simulink model "NewtonRaphson"  (R2018b)
settings: Solver=FixedStepAuto  StartTime=0.0  StopTime=10.0  FixedStep=1  RelTol=1e-3
undefined symbols (not defined in the file or in its folder): a, b, c
libraries: simulink x8, hdlsllib x3
settings Model: Creator=meyer  LastModifiedBy=meyer

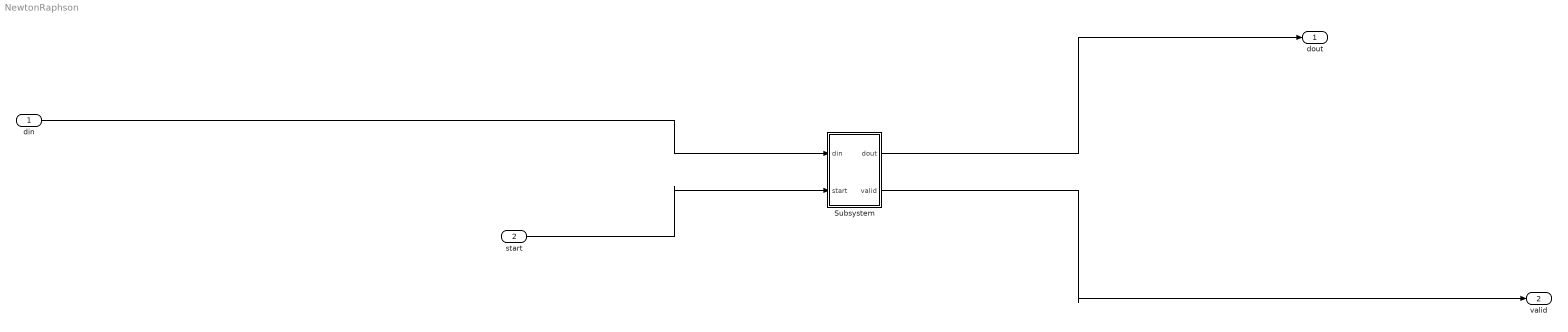
== system NewtonRaphson ==
  din : Inport  OutDataTypeStr=fixdt(1,32,16)
  start : Inport  Port=2  OutDataTypeStr=boolean
  Subsystem : Subsystem
  dout : Outport
  valid : Outport  Port=2
  wires:
  din/1 -> Subsystem/1(din)
  start/1 -> Subsystem/2(start)
  Subsystem/1(dout) -> dout/1
  Subsystem/2(valid) -> valid/1

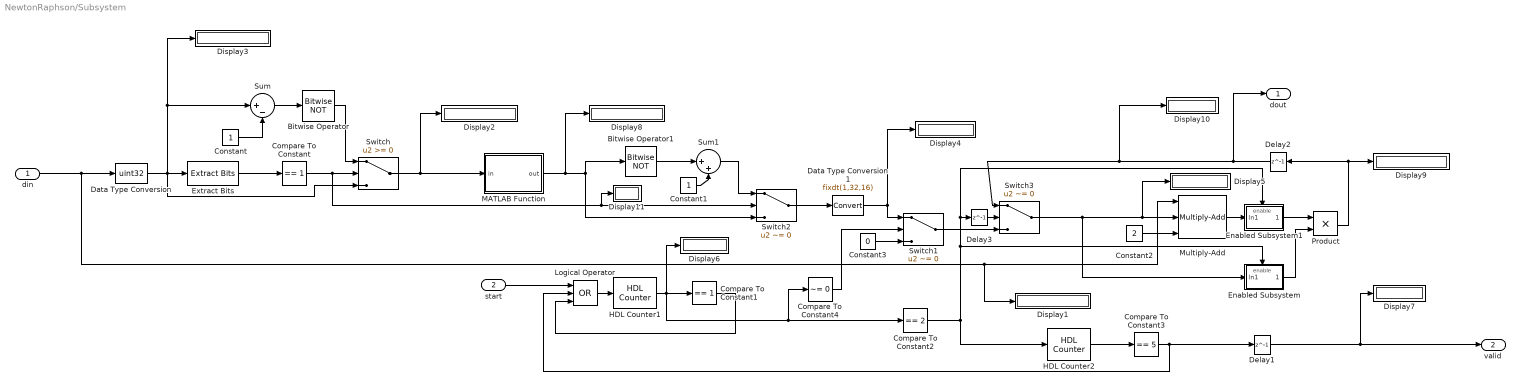
== system NewtonRaphson/Subsystem ==
  din : Inport  OutDataTypeStr=fixdt(1,32,16)
  start : Inport  Port=2  OutDataTypeStr=boolean
  Bitwise Operator : simulink/Logic and Bit Operations/Bitwise Operator  logicop=NOT  UseBitMask=off  BitMask=bin2dec('11011001')  BitMaskRealWorld=Stored Integer
  Bitwise Operator1 : simulink/Logic and Bit Operations/Bitwise Operator  logicop=NOT  UseBitMask=off  BitMask=bin2dec('11011001')  BitMaskRealWorld=Stored Integer
  Compare To Constant : simulink/Logic and Bit Operations/Compare To Constant  relop===  const=1  OutDataTypeStr=boolean
  Compare To Constant1 : simulink/Logic and Bit Operations/Compare To Constant  relop===  const=1  OutDataTypeStr=boolean
  Compare To Constant2 : simulink/Logic and Bit Operations/Compare To Constant  relop===  const=2  OutDataTypeStr=boolean
  Compare To Constant3 : simulink/Logic and Bit Operations/Compare To Constant  relop===  const=5  OutDataTypeStr=boolean
  Compare To Constant4 : simulink/Logic and Bit Operations/Compare To Constant  relop=~=  const=0  OutDataTypeStr=boolean
  Constant : Constant  OutDataTypeStr=uint32  SampleTime=-1
  Constant1 : Constant  OutDataTypeStr=uint32  SampleTime=-1
  Constant2 : Constant  Value=2  OutDataTypeStr=fixdt(1,32,16)  SampleTime=-1
  Constant3 : Constant  Value=0  OutDataTypeStr=fixdt(1,32,16)  SampleTime=-1
  Data Type Conversion : DataTypeConversion  OutDataTypeStr=uint32  ConvertRealWorld=Stored Integer (SI)
  Data Type Conversion1 : DataTypeConversion  OutDataTypeStr=fixdt(1,32,16)  ConvertRealWorld=Stored Integer (SI)
  Delay1 : Delay  DelayLength=1
  Delay2 : Delay  DelayLength=1
  Delay3 : Delay  DelayLength=1
  Display{1..11} (11 alike) : Display
      Display2 settings: Format=hex (Stored Integer)
      Display3 settings: Format=hex (Stored Integer)
      Display8 settings: Format=hex (Stored Integer)
  Enabled Subsystem : Subsystem  TreatAsAtomicUnit=on
  Enabled Subsystem1 : Subsystem  TreatAsAtomicUnit=on
  Extract Bits : simulink/Logic and Bit Operations/Extract Bits  bitsToExtract=Range of bits  numBits=1  bitIdxRange=31  outScalingMode=Treat bit field as an integer
      settings: SourceProductName=Simulink
  HDL Counter1 : hdlsllib/Sources/HDL Counter  CountType=Count limited  CountInit=0  CountStep=1  CountMax=2  CountFromType=Initial value  CountFrom=0  CountResetPort=off  CountLoadPort=off  CountEnbPort=on  CountDirPort=off  CountDataType=Unsigned  CountWordLen=4  CountFracLen=0  CountSampTime=1
      settings: SourceProductBaseCode=HD
  HDL Counter2 : hdlsllib/Sources/HDL Counter  CountType=Count limited  CountInit=0  CountStep=1  CountMax=5  CountFromType=Initial value  CountFrom=0  CountResetPort=off  CountLoadPort=off  CountEnbPort=on  CountDirPort=off  CountDataType=Unsigned  CountWordLen=4  CountFracLen=0  CountSampTime=1
      settings: SourceProductBaseCode=HD
  Logical Operator : Logic  Operator=OR  Inputs=3  IconShape=distinctive  AllPortsSameDT=off  OutDataTypeStr=boolean
  MATLAB Function : MATLAB Function
  Multiply-Add : hdlsllib/HDL Operations/Multiply-Add  Function=c-(a.*b)  datatype=fixdt(1,32,16)  DoSatur=off  FMA=off
      settings: SourceProductName=HDL Coder  SourceProductBaseCode=HD
  Product : Product  OutDataTypeStr=fixdt(1,32,16)
  Sum : Sum  Inputs=|+-
  Sum1 : Sum  Inputs=|++
  Switch : Switch
  Switch1 : Switch  Criteria=u2 ~= 0
  Switch2 : Switch  Criteria=u2 ~= 0  OutDataTypeStr=Inherit: Inherit via back propagation
  Switch3 : Switch  Criteria=u2 ~= 0
  dout : Outport
  valid : Outport  Port=2
  wires:
  Enabled Subsystem/1(Out1) -> Product/2
  MATLAB Function/1(out) -> Switch2/3, Bitwise Operator1/1, Display8/1
  HDL Counter1/1 -> Compare To Constant2/1, Compare To Constant4/1, Display6/1, Compare To Constant1/1
  Delay2/1 -> dout/1, Display10/1, Switch3/1
  Compare To Constant1/1 -> Logical Operator/3
  Compare To Constant/1 -> Display11/1, Switch2/2, Switch/2
  Constant1/1 -> Sum1/2
  Compare To Constant2/1 -> HDL Counter2/1, Enabled Subsystem1/Enable, Delay3/1, Enabled Subsystem/Enable
  Product/1 -> Delay2/1, Display9/1
  Multiply-Add/1 -> Enabled Subsystem1/1(In1)
  Compare To Constant3/1 -> Delay1/1, Logical Operator/2
  Switch1/1 -> Switch3/3
  start/1 -> Logical Operator/1
  Delay3/1 -> Switch3/2
  Constant3/1 -> Switch1/3
  Switch2/1 -> Data Type Conversion1/1
  Switch/1 -> Display2/1, MATLAB Function/1(in)
  Switch3/1 -> Display5/1, Multiply-Add/2, Enabled Subsystem/1(In1)
  Enabled Subsystem1/1(Out1) -> Product/1
  Sum/1 -> Bitwise Operator/1
  Constant/1 -> Sum/2
  Data Type Conversion1/1 -> Switch1/1, Display4/1
  Logical Operator/1 -> HDL Counter1/1
  Data Type Conversion/1 -> Switch/3, Extract Bits/1, Display3/1, Sum/1
  din/1 -> Multiply-Add/1, Display1/1, Data Type Conversion/1
  Bitwise Operator/1 -> Switch/1
  Extract Bits/1 -> Compare To Constant/1
  Constant2/1 -> Multiply-Add/3
  HDL Counter2/1 -> Compare To Constant3/1
  Delay1/1 -> valid/1, Display7/1
  Sum1/1 -> Switch2/1
  Compare To Constant4/1 -> Switch1/2
  Bitwise Operator1/1 -> Sum1/1

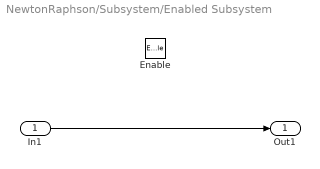
== system NewtonRaphson/Subsystem/Enabled Subsystem ==
  In1 : Inport
  Enable : EnablePort
  Out1 : Outport  InitialOutput=0
  wires:
  In1/1 -> Out1/1

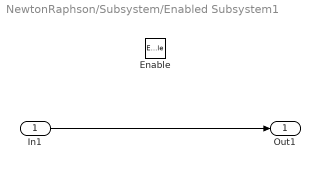
== system NewtonRaphson/Subsystem/Enabled Subsystem1 ==
  In1 : Inport
  Enable : EnablePort
  Out1 : Outport  InitialOutput=0
  wires:
  In1/1 -> Out1/1

== matlab function NewtonRaphson/Subsystem/MATLAB Function ==
  data: in input uint32; out output uint32
function out = fcn(in)
%#codegen

% Declare internal register
persistent out_i;
if isempty(out_i)
    out_i = uint32(0);
end

% Register output
out = out_i;

% Mux to get out_i
if bitget(in,31) == 1
    out_i = bitset(uint32(0), 2);
elseif bitget(in,30) == 1
    out_i = bitset(uint32(0), 3);
elseif bitget(in,29) == 1
    out_i = bitset(uint32(0), 4);
elseif bitget(in,28) == 1
    out_i = bitset(uint32(0), 5);
elseif bitget(in,27) == 1
    out_i = bitset(uint32(0), 6);
elseif bitget(in,26) == 1
    out_i = bitset(uint32(0), 7);
elseif bitget(in,25) == 1
    out_i = bitset(uint32(0), 8);
elseif bitget(in,24) == 1
    out_i = bitset(uint32(0), 9);
elseif bitget(in,23) == 1
    out_i = bitset(uint32(0), 10);
elseif bitget(in,22) == 1
    out_i = bitset(uint32(0), 11);
elseif bitget(in,21) == 1
    out_i = bitset(uint32(0), 12);
elseif bitget(in,20) == 1
    out_i = bitset(uint32(0), 13);
elseif bitget(in,19) == 1
    out_i = bitset(uint32(0), 14);
elseif bitget(in,18) == 1
    out_i = bitset(uint32(0), 15);
elseif bitget(in,17) == 1
    out_i = bitset(uint32(0), 16);
elseif bitget(in,16) == 1
    out_i = bitset(uint32(0), 17);
elseif bitget(in,15) == 1
    out_i = bitset(uint32(0), 18);
elseif bitget(in,14) == 1
    out_i = bitset(uint32(0), 19);
elseif bitget(in,13) == 1
    out_i = bitset(uint32(0), 20);
elseif bitget(in,12) == 1
    out_i = bitset(uint32(0), 21);
elseif bitget(in,11) == 1
    out_i = bitset(uint32(0), 22);
elseif bitget(in,10) == 1
    out_i = bitset(uint32(0), 23);
elseif bitget(in,9) == 1
    out_i = bitset(uint32(0), 24);
elseif bitget(in,8) == 1
    out_i = bitset(uint32(0), 25);
elseif bitget(in,7) == 1
    out_i = bitset(uint32(0), 26);
elseif bitget(in,6) == 1
    out_i = bitset(uint32(0), 27);
elseif bitget(in,5) == 1
    out_i = bitset(uint32(0), 28);
elseif bitget(in,4) == 1
    out_i = bitset(uint32(0), 29);
elseif bitget(in,3) == 1
    out_i = bitset(uint32(0), 30);
elseif bitget(in,2) == 1
    out_i = bitset(uint32(0), 31);
elseif bitget(in,1) == 1
    out_i = bitset(uint32(0), 32);
else
    out_i = uint32(0);
end

end
